simulink model "non_lin"  (R2022a)
settings: Solver=VariableStepAuto  StartTime=0.0  StopTime=T  RelTol=1e-3
values from neighbouring files (symbols this model uses):
  config = jsondecode(fileread(config_file_name))    [dh_analysis.m]    (also in init_klmn.m; static_ozf.m)
  hyb = dss(A_cal, [B1_cal, B2_cal], [C1_cal;C2_cal],[D11_cal, D12_cal;D21_cal,D22_cal], eye(2*nx), config.parameters.time_delta )    [static_ozf.m]
  nwp = size(config.parameters.B_lin, 2)    [dh_analysis.m]    (also in init_klmn.m; static_ozf.m)
  nwu = 5    [basic_klmn.m]    (also in dh_analysis.m = config.parameters.nwu; init_klmn.m = config.parameters.nwu; static_ozf.m = config.parameters.nwu)
  nx = size(A,1)    [basic_klmn.m]    (also in dh_analysis.m = size(config.parameters.A_lin, 1); init_klmn.m = size(config.parameters.A_lin, 1); static_ozf.m = size(config.parameters.A_lin, 1))
  nzu = nwu    (= 5)    [basic_klmn.m]    (also in dh_analysis.m = nwu; init_klmn.m = nwu; static_ozf.m = nwu)
settings Model: Creator=jack  LastModifiedBy=jack

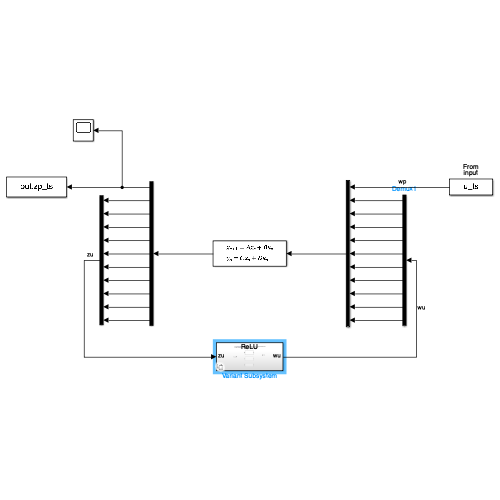
[thumbnail: Simulink's stored preview of the top-level diagram]
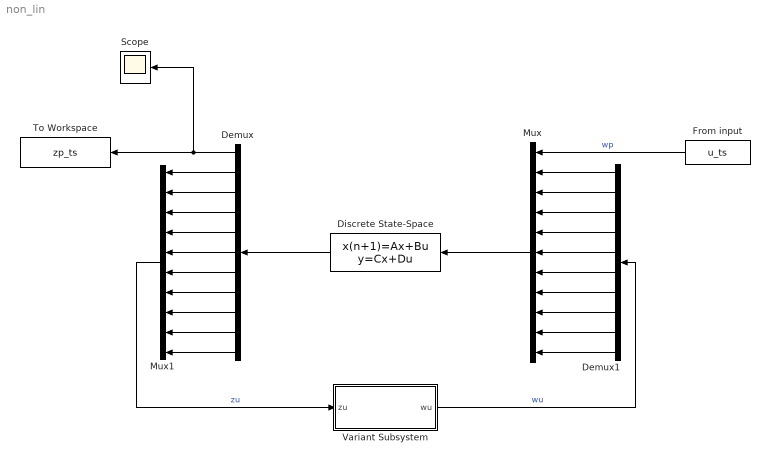
== system non_lin ==
  Demux : Demux  Outputs=nzu+nwp
  Demux1 : Demux  Outputs=nzu
  Discrete State-Space : DiscreteStateSpace  A=hyb.A  B=hyb.B  C=hyb.C  D=hyb.D  InitialCondition=zeros(2*nx,1)  SampleTime=config.parameters.time_delta
  From input : FromWorkspace  VariableName=u_ts  SampleTime=config.parameters.time_delta
  Mux : Mux  Inputs=nwu+nwp
  Mux1 : Mux  Inputs=nzu
  Scope : Scope
  To Workspace : ToWorkspace  VariableName=zp_ts  SaveFormat=Timeseries  SampleTime=-1
  Variant Subsystem : Subsystem  Variant=on
  wires:
  Discrete State-Space/1 -> Demux/1
  Mux/1 -> Discrete State-Space/1
  Demux/2 -> Mux1/1
  Demux/3 -> Mux1/2
  Demux/4 -> Mux1/3
  Demux/5 -> Mux1/4
  Demux/6 -> Mux1/5
  Demux/7 -> Mux1/6
  Demux/8 -> Mux1/7
  Demux/9 -> Mux1/8
  Demux/10 -> Mux1/9
  Demux/11 -> Mux1/10
  From input/1 -> Mux/1  "wp"
  Mux1/1 -> Variant Subsystem/1(zu)  "zu"
  Demux1/10 -> Mux/11
  Demux1/9 -> Mux/10
  Demux1/8 -> Mux/9
  Demux1/7 -> Mux/8
  Demux1/6 -> Mux/7
  Demux1/5 -> Mux/6
  Demux1/4 -> Mux/5
  Demux1/3 -> Mux/4
  Demux1/2 -> Mux/3
  Demux1/1 -> Mux/2
  Variant Subsystem/1(wu) -> Demux1/1  "wu"
  Demux/1 -> To Workspace/1, Scope/1

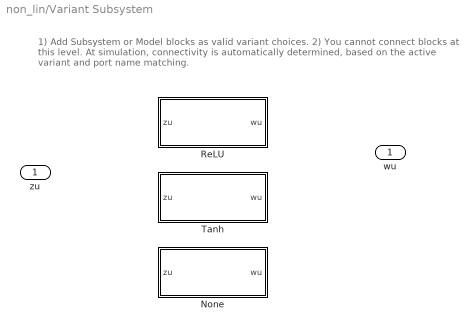
== system non_lin/Variant Subsystem ==
  note: 1) Add Subsystem or Model blocks as valid variant choices.
      | 2) You cannot connect blocks at this level. At simulation, connectivity is automatically
      | determined, based on the active variant and port name matching.
  zu : Inport
  None : Subsystem  VariantControl=nonlinearity == activation.None
  ReLU : Subsystem  VariantControl=nonlinearity == activation.ReLU
  Tanh : Subsystem  VariantControl=nonlinearity == activation.Tanh
  wu : Outport

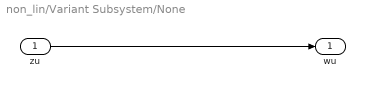
== system non_lin/Variant Subsystem/None ==
  zu : Inport
  wu : Outport
  wires:
  zu/1 -> wu/1

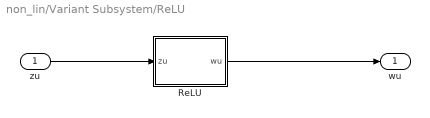
== system non_lin/Variant Subsystem/ReLU ==
  zu : Inport
  ReLU : MATLAB Function  TreatAsAtomicUnit=on  SystemSampleTime=config.parameters.time_delta
  wu : Outport
  wires:
  zu/1 -> ReLU/1(zu)
  ReLU/1(wu) -> wu/1

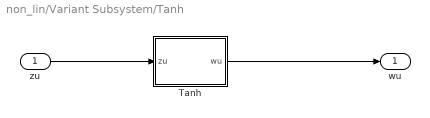
== system non_lin/Variant Subsystem/Tanh ==
  zu : Inport
  Tanh : MATLAB Function  TreatAsAtomicUnit=on  SystemSampleTime=config.parameters.time_delta
  wu : Outport
  wires:
  Tanh/1(wu) -> wu/1
  zu/1 -> Tanh/1(zu)

== matlab function non_lin/Variant Subsystem/Tanh/Tanh ==
  data: zu input; wu output
function wu = Tanh(zu)
wu = tanh(zu);

== matlab function non_lin/Variant Subsystem/ReLU/ReLU ==
  data: zu input; wu output
function wu = ReLU(zu)
wu = max(zu,0);
